simulink model "my_system"  (R2025b)
settings: Solver=ode15s  StartTime=0.0  StopTime=5  RelTol=1e-3
settings Model: Creator=user  LastModifiedBy=user

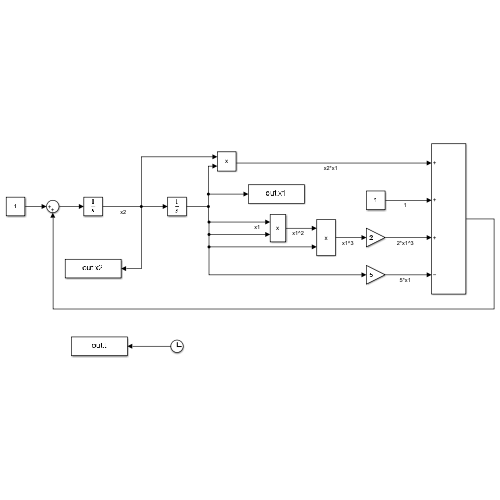
[thumbnail: Simulink's stored preview of the top-level diagram]
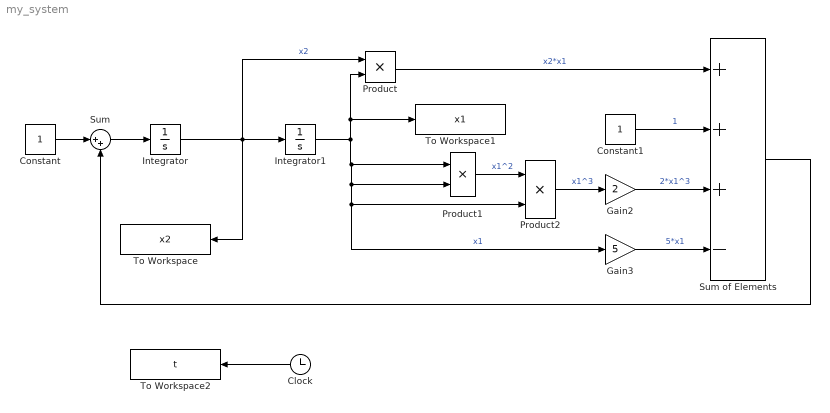
== system my_system ==
  Clock : Clock
  Constant : Constant
  Constant1 : Constant
  Gain2 : Gain  Gain=2
  Gain3 : Gain  Gain=5
  Integrator : Integrator  InitialCondition=0.001
  Integrator1 : Integrator  InitialCondition=0.001
  Product : Product
  Product1 : Product
  Product2 : Product
  Sum : Sum  Inputs=|++
  Sum of Elements : Sum  Inputs=+++-
  To Workspace : ToWorkspace  VariableName=x2  SampleTime=-1
  To Workspace1 : ToWorkspace  VariableName=x1  SampleTime=-1
  To Workspace2 : ToWorkspace  VariableName=t  SampleTime=-1
  wires:
  Integrator/1 -> To Workspace/1, Integrator1/1, Product/1  "x2"
  Constant/1 -> Sum/1
  Sum/1 -> Integrator/1
  Integrator1/1 -> Gain3/1, Product2/2, Product1/2, Product1/1, To Workspace1/1, Product/2  "x1"
  Product/1 -> Sum of Elements/1  "x2*x1"
  Product1/1 -> Product2/1  "x1^2"
  Product2/1 -> Gain2/1  "x1^3"
  Gain3/1 -> Sum of Elements/4  "5*x1"
  Gain2/1 -> Sum of Elements/3  "2*x1^3"
  Constant1/1 -> Sum of Elements/2  "1"
  Sum of Elements/1 -> Sum/2
  Clock/1 -> To Workspace2/1
